simulink model "EngReq_TrqLimCalc"  (R2018a)
settings: configuration reference "cs_ert" (kept outside this file)
settings Model: DataDictionary=EngReq_TrqLimCalc.sldd  Creator=zhoutinglin  LastModifiedBy=zhoutinglin

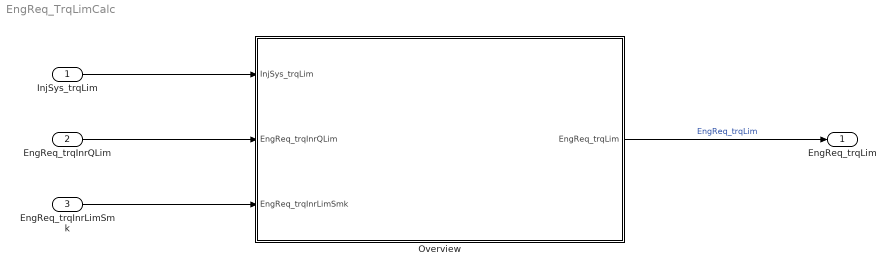
== system EngReq_TrqLimCalc ==
  InjSys_trqLim : Inport  Description=Torque limitation of injection system  OutMin=-3276.8  OutMax=3276.7  OutDataTypeStr=Torq  Unit=Nm  PortDimensions=[1 1]
  EngReq_trqInrQLim : Inport  Description=Limiting torque due to limitation quantities (except smoke limitation)  Port=2  OutMin=-3276.8  OutMax=3276.7  OutDataTypeStr=Torq  Unit=Nm  PortDimensions=[1 1]
  EngReq_trqInrLimSmk : Inport  Description=Limiting torque smoke limit  Port=3  OutMin=-3276.8  OutMax=3276.7  OutDataTypeStr=Torq  Unit=Nm  PortDimensions=[1 1]
  Overview : Subsystem
  EngReq_trqLim : Outport
  wires:
  InjSys_trqLim/1 -> Overview/1(InjSys_trqLim)
  EngReq_trqInrQLim/1 -> Overview/2(EngReq_trqInrQLim)
  EngReq_trqInrLimSmk/1 -> Overview/3(EngReq_trqInrLimSmk)
  Overview/1(EngReq_trqLim) -> EngReq_trqLim/1  "EngReq_trqLim"

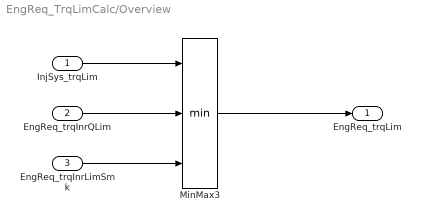
== system EngReq_TrqLimCalc/Overview ==
  InjSys_trqLim : Inport  Tag=Nm
  EngReq_trqInrQLim : Inport  Tag=Nm  Port=2
  EngReq_trqInrLimSmk : Inport  Tag=Nm  Port=3
  MinMax3 : MinMax  Inputs=3  InputSameDT=on
  EngReq_trqLim : Outport  Tag=Nm
  wires:
  EngReq_trqInrQLim/1 -> MinMax3/2
  InjSys_trqLim/1 -> MinMax3/1
  MinMax3/1 -> EngReq_trqLim/1
  EngReq_trqInrLimSmk/1 -> MinMax3/3
